simulink library "ddm"  (R2021b)
settings: Solver=VariableStepAuto  StartTime=0.0  StopTime=10.0  RelTol=1e-3
undefined symbols (not defined in the file or in its folder): ENUM_ADASACCSTA_ERROR, ENUM_ADASACCSTA_OFF, ENUM_ADASACCSTA_STANDBY, ENUM_ADASISASTA_OFF, ENUM_ALLOWMOV_ALLOWREADY, ENUM_APS, ENUM_BRKSTA_ERROR, ENUM_BRKSTA_OFF, ENUM_BRKSTA_ON, ENUM_CHGPREACTERRSTA_OBCPRE, ENUM_DCDCFAULTSTA_ANYFAULTLV1, ENUM_DCDCFAULTSTA_ANYFAULTLV2, ENUM_DRIVETRAIN_AWD, ENUM_DRIVETRAIN_FWD, ENUM_DRIVETRAIN_RWD, ENUM_DRSEATSTA_INVALID, ENUM_EDUDRTSTA_NORMAL, ENUM_EPBSTA_APPLIED, ENUM_EPBSTA_RELEASED, ENUM_HVBATTREADYPRE_READY, ENUM_MCUWARN_LV0, ENUM_MCUWARN_LV1, ENUM_MCUWARN_LV2, ENUM_MCUWARN_LV3, ENUM_MCUWARN_NOERROR, ENUM_OBCFAULTSTA_ANYFAULT, ENUM_PAS_R2F2, ENUM_PDFAULT_BATTPDFAIL, ENUM_PDFAULT_DCDCDISABLE, ENUM_PDFAULT_MCUDISABLE, ENUM_PDFAULT_MCUDISCHRG, ENUM_POWERSTA_OFF, ENUM_POWERSTA_ON, ENUM_POWERSTA_READY, ENUM_POWERSTA_STANDBY, ENUM_PRESSINDI_LOW, ENUM_PUFAULT_BATTUPFAIL, ENUM_PUFAULT_DCDCENABLEFAIL, ENUM_PUFAULT_PRECHRGCHKFAIL, ENUM_PUFAULT_SAFETYCHKFAIL, ENUM_PUSTATE_COMPLETED, ENUM_PWRSTASW_OFF, ENUM_PWRSTASW_OFFA, ENUM_PWRSTASW_OFFCHVCHRG, ENUM_PWRSTASW_OFFCLVCHRG, ENUM_PWRSTASW_ON, ENUM_PWRSTASW_ONHVCHRG, ENUM_PWRSTASW_READY, ENUM_PWRSTASW_STANDBY, ENUM_RANGESTA_12IN, ENUM_RANGESTA_12OUT, ENUM_SHIFTCOMMAND_D, ENUM_SHIFTCOMMAND_N, ENUM_SHIFTCOMMAND_P, ENUM_SHIFTCOMMAND_R, ENUM_ZONEMALFUNLV_1ST, ENUM_ZONEMALFUNLV_2ND, ENUM_ZONEMALFUNLV_3RD, ENUM_ZONEMALFUNLV_4TH, ENUM_ZONESPDCTRLMODE_ACC ... (+832)
libraries: hcu_lib x738, $bdroot x26, simulink x7
(part 19 of 25)

== system ddm/DDM/DDM/PMM/power up and power down/HVB ready for precharge fail ==
  note: Fail Safe Operation After Failure Decision
  note: Diagnostics and Fault Handling
  note: Release Condition After Failure Decision
  note: Fail Safe Operation During Failure Detection
  note: Test Pass Criteria
  note: Test Detection Criteria
  note: Release Condition During Failure Detection
  task_time_s : Inport
  VPMM_PowerSta_enum : Inport  Port=2
  VPMM_PwrStaSW_enum : Inport  Port=3
  VINP_HVBattReady4Pre_enum : Inport  Port=4
  VPMM_PowerUpFault_enum : Inport  Port=5
  DTC_clear_request : Inport  Port=6
  VPMM_PowerUpState_enum : Inport  Port=7
  Constant : Constant  Value=ENUM_PUFAULT_PRECHRGCHKFAIL
  Constant1 : Constant  Value=ENUM_PUSTATE_COMPLETED
  Constant10 : Constant  Value=KDDM_HVB4PreDTC_cnt
  Constant11 : Constant  Value=KDDM_HVB4PrePassSW_flg
  Constant15 : Constant  Value=KDDM_HVB4PreCFSSW_flg
  Constant16 : Constant  Value=TRUE
  Constant19 : Constant  Value=ENUM_POWERSTA_OFF
  Constant{2,21,25,27} (4 alike) : Constant  Value=FALSE
  Constant20 : Constant  Value=KDDM_HVB4PreDFSSW_flg
  Constant23 : Constant  Value=TRUE
  Constant24 : Constant  Value=TRUE
  Constant26 : Constant  Value=ENUM_PWRSTASW_OFF
  Constant3 : Constant  Value=ENUM_HVBATTREADYPRE_READY
  Constant38 : Constant  Commented=on  Value=KDDM_HVB4PreDetTO_s
  Constant40 : Constant  Commented=on  Value=KDDM_HVB4PreDTC_cnt
  Constant43 : Constant  Value=KDDM_HVB4PrePassTO_s
  Constant44 : Constant  Value=KDDM_HVB4PreDetSW_flg
  Constant8 : Constant  Value=KDDM_HVB4PrePassTO_s
  DTC_Couter : hcu_lib/Basic_Blocks/DTC_Couter
  DTC_Info : hcu_lib/Basic_Blocks/DTC_Info
  Data Type Conversion1 : DataTypeConversion  OutDataTypeStr=uint8
  Equal : RelationalOperator  Operator=~=  OutDataTypeStr=boolean  RndMeth=Simplest
  Equal1 : RelationalOperator  Operator===  OutDataTypeStr=boolean  RndMeth=Simplest
  Equal24 : RelationalOperator  Operator=~=  OutDataTypeStr=boolean  RndMeth=Simplest
  Equal4 : RelationalOperator  OutDataTypeStr=boolean  RndMeth=Simplest
  Equal5 : RelationalOperator  Operator===  OutDataTypeStr=boolean  RndMeth=Simplest
  Equal8 : RelationalOperator  Operator===  OutDataTypeStr=boolean  RndMeth=Simplest
  From48 : From  Commented=on  GotoTag=task_time_s
  Goto24 : Goto  Commented=on  GotoTag=VDDM_EDriveSysErrVCUErr_flg
  Logical Operator{4,12,15,18..19} (5 alike) : Logic  AllPortsSameDT=off  OutDataTypeStr=boolean
  Logical Operator3 : Logic  Operator=OR  AllPortsSameDT=off  OutDataTypeStr=boolean
  Logical Operator6 : Logic  Operator=NOT  AllPortsSameDT=off  OutDataTypeStr=boolean
  Logical Operator8 : Logic  Operator=OR  AllPortsSameDT=off  OutDataTypeStr=boolean
  Relay : Relay  OnSwitchValue=ONE_INT  OffSwitchValue=ZERO_INT
  SR_Latch1 : Subsystem  mask(SR_Latch){}
      mask help: SR latch function.
  SR_Latch3 : hcu_lib/Basic_Blocks/SR_Latch
  SR_Latch4 : hcu_lib/Basic_Blocks/SR_Latch
  Switch{,2,4..5} (4 alike) : Switch  Criteria=u2 ~= 0
  Test Detection Criteria : hcu_lib/Basic_Blocks/Test Detection Criteria  Commented=on
  Timer1 : hcu_lib/Basic_Blocks/Timer
  VDDM_HVB4PreDTC_raw32 : Outport
  wires:
  VPMM_PowerSta_enum/1 -> [VPMM_PowerSta_enum]
  VPMM_PwrStaSW_enum/1 -> [VPMM_PwrStaSW_enum]
  task_time_s/1 -> [task_time_s]
  Constant3/1 -> Equal24/2
  VINP_HVBattReady4Pre_enum/1 -> Equal24/1
  Logical Operator15/1 -> DTC_Couter/2
  Data Type Conversion1/1 -> [VDDM_HVB4PreDTC_cnt]  "VDDM_HVB4PreDTC_cnt"
  Constant11/1 -> Logical Operator15/2
  Constant40/1 -> Test Detection Criteria/3
  Constant43/1 -> Timer1/4
  Switch5/1 -> [VDDM_HVB4PreDet_flg]  "VDDM_HVB4PreDet_flg"
  Logical Operator3/1 -> Logical Operator15/1
  [VDDM_HVB4PreDTC_cnt] -> Relay/1
  [DTC_clear_request] -> Logical Operator8/2
  Constant23/1 -> Switch2/3
  Constant8/1 -> Equal4/2
  SR_Latch4/1 -> Logical Operator18/1
  Constant25/1 -> Switch4/3
  [VDDM_HVB4PreDet_flg] -> Logical Operator19/1
  Constant20/1 -> Logical Operator12/1
  Constant21/1 -> Switch/3
  Equal4/1 -> SR_Latch1/1(set)
  Switch4/1 -> [VDDM_HVB4PreCFSRls_flg]
  Constant26/1 -> Equal/2
  Logical Operator8/1 -> Switch4/2
  Constant16/1 -> Switch/1
  [VPMM_PowerSta_enum] -> Equal5/1
  Switch/1 -> Goto24/1
  SR_Latch3/1 -> Logical Operator12/2
  [VDDM_HVB4PreCFSRls_flg] -> Logical Operator3/2
  Logical Operator18/1 -> [VDDM_HVB4PreCFS_flg]
  DTC_Couter/2 -> Data Type Conversion1/1
  [VDDM_HVB4PrePass_flg] -> Logical Operator3/1
  Switch2/1 -> SR_Latch1/2(reset), Timer1/2, Logical Operator6/1
  Constant15/1 -> Logical Operator18/2
  Equal/1 -> Switch5/2
  Relay/1 -> SR_Latch3/1
  From48/1 -> Test Detection Criteria/2
  Logical Operator19/1 -> DTC_Couter/1
  [VDDM_HVB4PreCFS_flg] -> Switch/2
  [VPMM_PwrStaSW_enum] -> Equal/1
  Constant24/1 -> Switch4/1
  DTC_Couter/1 -> SR_Latch4/1
  SR_Latch1/1(latched) -> [VDDM_HVB4PrePass_flg]
  Logical Operator12/1 -> [VDDM_HVB4PreDFS_flg]
  Logical Operator6/1 -> Timer1/1
  Constant19/1 -> Equal5/2
  Constant27/1 -> Switch5/3
  Constant44/1 -> Logical Operator19/2
  Timer1/1 -> Equal4/1
  Equal5/1 -> Logical Operator8/1
  [VDDM_HVB4PreCFSRls_flg] -> SR_Latch4/2
  Constant10/1 -> DTC_Couter/3
  [VDDM_HVB4PreChk_flg] -> Switch5/1
  Constant1/1 -> Equal1/2
  Constant2/1 -> Switch2/1
  [VPMM_PowerUpState_enum] -> Equal1/1
  DTC_clear_request/1 -> [DTC_clear_request]
  Constant/1 -> Equal8/2
  VPMM_PowerUpFault_enum/1 -> Equal8/1
  Equal24/1 -> Logical Operator4/1
  Equal8/1 -> Logical Operator4/2
  Logical Operator4/1 -> [VDDM_HVB4PreChk_flg]
  [task_time_s] -> Timer1/3
  Equal1/1 -> Switch2/2
  DTC_Info/1 -> VDDM_HVB4PreDTC_raw32/1  "VDDM_HVB4PreDTC_raw32"
  [VDDM_HVB4PreCFS_flg] -> DTC_Info/3
  [VDDM_HVB4PreCFS_flg] -> SR_Latch3/2
  [VDDM_HVB4PrePass_flg] -> DTC_Info/2
  [VDDM_HVB4PreDet_flg] -> DTC_Info/1
  Constant38/1 -> Test Detection Criteria/4
  [DTC_clear_request] -> DTC_Info/4
  VPMM_PowerUpState_enum/1 -> [VPMM_PowerUpState_enum]

== system ddm/DDM/DDM/PMM/power up and power down/High level system safety check fail ==
  note: Fail Safe Operation After Failure Decision
  note: Fail Safe Operation During Failure Detection
  note: Diagnostics and Fault Handling
  note: Release Condition During Failure Detection
  note: Test Pass Criteria
  note: Test Detection Criteria
  note: Release Condition After Failure Decision
  task_time_s : Inport
  VPMM_PowerSta_enum : Inport  Port=2
  VPMM_PwrStaSW_enum : Inport  Port=3
  VPMM_SafetyChkHLv_flg : Inport  Port=4
  VPMM_PowerUpFault_enum : Inport  Port=5
  DTC_clear_request : Inport  Port=6
  VPMM_PowerUpState_enum : Inport  Port=7
  Constant : Constant  Value=ENUM_PUFAULT_SAFETYCHKFAIL
  Constant1 : Constant  Value=ENUM_PUSTATE_COMPLETED
  Constant10 : Constant  Value=KDDM_HiLvSaChkDTC_cnt
  Constant11 : Constant  Value=KDDM_HiLvSaChkPassSW_flg
  Constant15 : Constant  Value=KDDM_HiLvSaChkCFSSW_flg
  Constant16 : Constant  Value=TRUE
  Constant19 : Constant  Value=ENUM_POWERSTA_OFF
  Constant{2,21,25,27} (4 alike) : Constant  Value=FALSE
  Constant20 : Constant  Value=KDDM_HiLvSaChkDFSSW_flg
  Constant23 : Constant  Value=TRUE
  Constant24 : Constant  Value=TRUE
  Constant26 : Constant  Value=ENUM_PWRSTASW_OFF
  Constant38 : Constant  Commented=on  Value=KDDM_HiLvSaChkDetTO_s
  Constant40 : Constant  Commented=on  Value=KDDM_HiLvSaChkDTC_cnt
  Constant43 : Constant  Value=KDDM_HiLvSaChkPassTO_s
  Constant44 : Constant  Value=KDDM_HiLvSaChkDetSW_flg
  Constant8 : Constant  Value=KDDM_HiLvSaChkPassTO_s
  DTC_Couter : hcu_lib/Basic_Blocks/DTC_Couter
  DTC_Info : hcu_lib/Basic_Blocks/DTC_Info
  Data Type Conversion1 : DataTypeConversion  OutDataTypeStr=uint8
  Equal : RelationalOperator  Operator=~=  OutDataTypeStr=boolean  RndMeth=Simplest
  Equal1 : RelationalOperator  Operator===  OutDataTypeStr=boolean  RndMeth=Simplest
  Equal2 : RelationalOperator  Operator===  OutDataTypeStr=boolean  RndMeth=Simplest
  Equal5 : RelationalOperator  OutDataTypeStr=boolean  RndMeth=Simplest
  Equal6 : RelationalOperator  Operator===  OutDataTypeStr=boolean  RndMeth=Simplest
  From48 : From  Commented=on  GotoTag=task_time_s
  Goto24 : Goto  Commented=on  GotoTag=VDDM_EDriveSysErrVCUErr_flg
  Logical Operator{5,12,15,18..19} (5 alike) : Logic  AllPortsSameDT=off  OutDataTypeStr=boolean
  Logical Operator3 : Logic  Operator=OR  AllPortsSameDT=off  OutDataTypeStr=boolean
  Logical Operator4 : Logic  Operator=NOT  AllPortsSameDT=off  OutDataTypeStr=boolean
  Logical Operator6 : Logic  Operator=NOT  AllPortsSameDT=off  OutDataTypeStr=boolean
  Logical Operator8 : Logic  Operator=OR  AllPortsSameDT=off  OutDataTypeStr=boolean
  Relay : Relay  OnSwitchValue=ONE_INT  OffSwitchValue=ZERO_INT
  SR_Latch1 : Subsystem  mask(SR_Latch){}
      mask help: SR latch function.
  SR_Latch3 : hcu_lib/Basic_Blocks/SR_Latch
  SR_Latch4 : hcu_lib/Basic_Blocks/SR_Latch
  Switch{,2,4..5} (4 alike) : Switch  Criteria=u2 ~= 0
  Test Detection Criteria : hcu_lib/Basic_Blocks/Test Detection Criteria  Commented=on
  Timer1 : hcu_lib/Basic_Blocks/Timer
  VDDM_HiLvSaChkDTC_raw32 : Outport
  wires:
  Logical Operator5/1 -> [VDDM_HiLvSaChkChk_flg]
  VPMM_PowerUpFault_enum/1 -> Equal1/1
  VPMM_SafetyChkHLv_flg/1 -> Logical Operator4/1
  Logical Operator4/1 -> Logical Operator5/1
  Equal1/1 -> Logical Operator5/2
  Constant/1 -> Equal1/2
  DTC_clear_request/1 -> [DTC_clear_request]
  [VDDM_HiLvSaChkCFSRls_flg] -> SR_Latch4/2
  Switch2/1 -> Logical Operator6/1, Timer1/2, SR_Latch1/2(reset)
  Timer1/1 -> Equal5/1
  [VDDM_HiLvSaChkChk_flg] -> Switch5/1
  Constant19/1 -> Equal6/2
  Constant44/1 -> Logical Operator19/2
  DTC_Couter/2 -> Data Type Conversion1/1
  Constant43/1 -> Timer1/4
  Constant27/1 -> Switch5/3
  Equal6/1 -> Logical Operator8/1
  SR_Latch1/1(latched) -> [VDDM_HiLvSaChkPass_flg]
  Logical Operator6/1 -> Timer1/1
  Logical Operator8/1 -> Switch4/2
  Equal/1 -> Switch5/2
  Equal2/1 -> Switch2/2
  [VDDM_HiLvSaChkDTC_cnt] -> Relay/1
  Constant11/1 -> Logical Operator15/2
  [DTC_clear_request] -> Logical Operator8/2
  [VDDM_HiLvSaChkCFS_flg] -> Switch/2
  Relay/1 -> SR_Latch3/1
  [VPMM_PwrStaSW_enum] -> Equal/1
  Constant25/1 -> Switch4/3
  Constant40/1 -> Test Detection Criteria/3
  Constant10/1 -> DTC_Couter/3
  Logical Operator15/1 -> DTC_Couter/2
  SR_Latch4/1 -> Logical Operator18/1
  Constant24/1 -> Switch4/1
  Logical Operator3/1 -> Logical Operator15/1
  [VDDM_HiLvSaChkDet_flg] -> Logical Operator19/1
  Switch5/1 -> [VDDM_HiLvSaChkDet_flg]  "VDDM_HiLvSaChkDet_flg"
  Switch/1 -> Goto24/1
  From48/1 -> Test Detection Criteria/2
  SR_Latch3/1 -> Logical Operator12/2
  Constant26/1 -> Equal/2
  Constant16/1 -> Switch/1
  Constant23/1 -> Switch2/3
  [VDDM_HiLvSaChkPass_flg] -> Logical Operator3/1
  [VPMM_PowerSta_enum] -> Equal6/1
  Logical Operator19/1 -> DTC_Couter/1
  [VDDM_HiLvSaChkCFSRls_flg] -> Logical Operator3/2
  DTC_Couter/1 -> SR_Latch4/1
  [task_time_s] -> Timer1/3
  Constant15/1 -> Logical Operator18/2
  Logical Operator12/1 -> [VDDM_HiLvSaChkDFS_flg]
  Constant20/1 -> Logical Operator12/1
  Constant8/1 -> Equal5/2
  Data Type Conversion1/1 -> [VDDM_HiLvSaChkDTC_cnt]  "VDDM_HiLvSaChkDTC_cnt"
  Switch4/1 -> [VDDM_HiLvSaChkCFSRls_flg]
  Equal5/1 -> SR_Latch1/1(set)
  Constant21/1 -> Switch/3
  Logical Operator18/1 -> [VDDM_HiLvSaChkCFS_flg]
  VPMM_PowerSta_enum/1 -> [VPMM_PowerSta_enum]
  VPMM_PwrStaSW_enum/1 -> [VPMM_PwrStaSW_enum]
  task_time_s/1 -> [task_time_s]
  DTC_Info/1 -> VDDM_HiLvSaChkDTC_raw32/1  "VDDM_HiLvSaChkDTC_raw32"
  [VDDM_HiLvSaChkPass_flg] -> DTC_Info/2
  [VDDM_HiLvSaChkCFS_flg] -> DTC_Info/3
  [VDDM_HiLvSaChkCFS_flg] -> SR_Latch3/2
  [VDDM_HiLvSaChkDet_flg] -> DTC_Info/1
  Constant38/1 -> Test Detection Criteria/4
  [DTC_clear_request] -> DTC_Info/4
  VPMM_PowerUpState_enum/1 -> [VPMM_PowerUpState_enum]
  Constant2/1 -> Switch2/1
  Constant1/1 -> Equal2/2
  [VPMM_PowerUpState_enum] -> Equal2/1

== system ddm/DDM/DDM/PMM/power up and power down/MCU active discharge fail ==
  note: Release Condition During Failure Detection
  note: Fail Safe Operation After Failure Decision
  note: Fail Safe Operation During Failure Detection
  note: Test Detection Criteria
  note: Diagnostics and Fault Handling
  note: Test Pass Criteria
  note: Release Condition After Failure Decision
  task_time_s : Inport
  VPMM_PowerSta_enum : Inport  Port=2
  VPMM_PwrStaSW_enum : Inport  Port=3
  VPMM_PowerDownFault_enum : Inport  Port=4
  DTC_clear_request : Inport  Port=5
  Constant : Constant  Value=ENUM_PDFAULT_MCUDISCHRG
  Constant1 : Constant  Value=ENUM_PWRSTASW_OFF
  Constant10 : Constant  Value=KDDM_MCUActDTC_cnt
  Constant11 : Constant  Value=KDDM_MCUActPassSW_flg
  Constant15 : Constant  Value=KDDM_MCUActCFSSW_flg
  Constant16 : Constant  Value=TRUE
  Constant17 : Constant  Value=KDDM_MCUActPassTO_s
  Constant19 : Constant  Value=ENUM_POWERSTA_OFF
  Constant20 : Constant  Value=KDDM_MCUActDFSSW_flg
  Constant21 : Constant  Value=FALSE
  Constant22 : Constant  Value=ENUM_PWRSTASW_OFF
  Constant23 : Constant  Value=TRUE
  Constant24 : Constant  Value=TRUE
  Constant25 : Constant  Value=FALSE
  Constant27 : Constant  Value=FALSE
  Constant38 : Constant  Commented=on  Value=KDDM_MCUActDetTO_s
  Constant40 : Constant  Commented=on  Value=KDDM_MCUActDTC_cnt
  Constant43 : Constant  Value=KDDM_MCUActPassTO_s
  Constant44 : Constant  Value=KDDM_MCUActDetSW_flg
  DTC_Couter : hcu_lib/Basic_Blocks/DTC_Couter
  DTC_Info : hcu_lib/Basic_Blocks/DTC_Info
  Data Type Conversion1 : DataTypeConversion  OutDataTypeStr=uint8
  Equal1 : RelationalOperator  Operator===  OutDataTypeStr=boolean  RndMeth=Simplest
  Equal2 : RelationalOperator  Operator=~=  OutDataTypeStr=boolean  RndMeth=Simplest
  Equal4 : RelationalOperator  Operator=~=  OutDataTypeStr=boolean  RndMeth=Simplest
  Equal6 : RelationalOperator  OutDataTypeStr=boolean  RndMeth=Simplest
  Equal7 : RelationalOperator  Operator===  OutDataTypeStr=boolean  RndMeth=Simplest
  From48 : From  Commented=on  GotoTag=task_time_s
  Logical Operator{12,15,18..19} (4 alike) : Logic  AllPortsSameDT=off  OutDataTypeStr=boolean
  Logical Operator3 : Logic  Operator=OR  AllPortsSameDT=off  OutDataTypeStr=boolean
  Logical Operator6 : Logic  Operator=NOT  AllPortsSameDT=off  OutDataTypeStr=boolean
  Logical Operator8 : Logic  Operator=OR  AllPortsSameDT=off  OutDataTypeStr=boolean
  Relay : Relay  OnSwitchValue=ONE_INT  OffSwitchValue=ZERO_INT
  SR_Latch1 : Subsystem  mask(SR_Latch){}
      mask help: SR latch function.
  SR_Latch3 : hcu_lib/Basic_Blocks/SR_Latch
  SR_Latch4 : hcu_lib/Basic_Blocks/SR_Latch
  Switch{,1,4..5} (4 alike) : Switch  Criteria=u2 ~= 0
  Test Detection Criteria : hcu_lib/Basic_Blocks/Test Detection Criteria  Commented=on
  Timer1 : hcu_lib/Basic_Blocks/Timer
  VDDM_MCUActDTC_raw32 : Outport
  VDDM_MCUActDisFail_flg : Outport  Port=2
  wires:
  VPMM_PowerSta_enum/1 -> [VPMM_PowerSta_enum]
  VPMM_PwrStaSW_enum/1 -> [VPMM_PwrStaSW_enum]
  task_time_s/1 -> [task_time_s]
  DTC_Couter/1 -> SR_Latch4/1
  Constant27/1 -> Switch5/3
  Constant23/1 -> Switch1/3
  SR_Latch4/1 -> Logical Operator18/1
  Constant11/1 -> Logical Operator15/2
  [VPMM_PowerSta_enum] -> Equal7/1
  Logical Operator15/1 -> DTC_Couter/2
  Constant20/1 -> Logical Operator12/1
  Equal2/1 -> Switch1/2
  [VDDM_MCUActDTC_cnt] -> Relay/1
  SR_Latch1/1(latched) -> [VDDM_MCUActPass_flg]
  Equal4/1 -> Switch5/2
  [VPMM_PwrStaSW_enum] -> Equal2/1
  Logical Operator12/1 -> [VDDM_MCUActDFS_flg]
  Constant1/1 -> Equal2/2
  Switch5/1 -> [VDDM_MCUActDet_flg]  "VDDM_MCUActDet_flg"
  Constant15/1 -> Logical Operator18/2
  [DTC_clear_request] -> Logical Operator8/2
  Constant40/1 -> Test Detection Criteria/3
  Switch4/1 -> [VDDM_MCUActCFSRls_flg]
  From48/1 -> Test Detection Criteria/2
  [VDDM_MCUActCFSRls_flg] -> Logical Operator3/2
  DTC_Couter/2 -> Data Type Conversion1/1
  SR_Latch3/1 -> Logical Operator12/2
  Constant17/1 -> Equal6/2
  Data Type Conversion1/1 -> [VDDM_MCUActDTC_cnt]  "VDDM_MCUActDTC_cnt"
  Logical Operator6/1 -> Timer1/1
  Switch/1 -> [VDDM_MCUActDisFail_flg]  "VDDM_MCUActDisFail_flg"
  Constant24/1 -> Switch4/1
  Constant16/1 -> Switch/1
  Timer1/1 -> Equal6/1
  Logical Operator18/1 -> [VDDM_MCUActCFS_flg]
  Switch1/1 -> Logical Operator6/1, SR_Latch1/2(reset), Timer1/2
  Constant10/1 -> DTC_Couter/3
  Logical Operator19/1 -> DTC_Couter/1
  Equal6/1 -> SR_Latch1/1(set)
  Constant44/1 -> Logical Operator19/2
  Constant43/1 -> Timer1/4
  Relay/1 -> SR_Latch3/1
  Logical Operator8/1 -> Switch4/2
  Constant22/1 -> Equal4/2
  Constant25/1 -> Switch4/3
  Equal7/1 -> Logical Operator8/1
  [VDDM_MCUActChk_flg] -> Switch1/1
  [VDDM_MCUActCFSRls_flg] -> SR_Latch4/2
  [VDDM_MCUActCFS_flg] -> Switch/2
  [task_time_s] -> Timer1/3
  Constant21/1 -> Switch/3
  [VPMM_PwrStaSW_enum] -> Equal4/1
  Logical Operator3/1 -> Logical Operator15/1
  [VDDM_MCUActPass_flg] -> Logical Operator3/1
  [VDDM_MCUActDet_flg] -> Logical Operator19/1
  Constant19/1 -> Equal7/2
  [VDDM_MCUActChk_flg] -> Switch5/1
  DTC_clear_request/1 -> [DTC_clear_request]
  Constant/1 -> Equal1/2
  VPMM_PowerDownFault_enum/1 -> Equal1/1
  Equal1/1 -> [VDDM_MCUActChk_flg]
  [VDDM_MCUActDisFail_flg] -> VDDM_MCUActDisFail_flg/1
  DTC_Info/1 -> VDDM_MCUActDTC_raw32/1  "VDDM_MCUActDTC_raw32"
  [VDDM_MCUActPass_flg] -> DTC_Info/2
  [VDDM_MCUActCFS_flg] -> DTC_Info/3
  [VDDM_MCUActCFS_flg] -> SR_Latch3/2
  [VDDM_MCUActDet_flg] -> DTC_Info/1
  Constant38/1 -> Test Detection Criteria/4
  [DTC_clear_request] -> DTC_Info/4

== system ddm/DDM/DDM/PMM/power up and power down/MCU disable fail ==
  note: Test Pass Criteria
  note: Release Condition After Failure Decision
  note: Test Detection Criteria
  note: Fail Safe Operation During Failure Detection
  note: Diagnostics and Fault Handling
  note: Release Condition During Failure Detection
  note: Fail Safe Operation After Failure Decision
  task_time_s : Inport
  VPMM_PowerSta_enum : Inport  Port=2
  VPMM_PwrStaSW_enum : Inport  Port=3
  VPMM_PowerDownFault_enum : Inport  Port=4
  DTC_clear_request : Inport  Port=5
  Constant : Constant  Value=ENUM_PDFAULT_MCUDISABLE
  Constant10 : Constant  Value=KDDM_MCUDisDTC_cnt
  Constant11 : Constant  Value=KDDM_MCUDisPassSW_flg
  Constant15 : Constant  Value=KDDM_MCUDisCFSSW_flg
  Constant16 : Constant  Value=TRUE
  Constant17 : Constant  Value=KDDM_MCUDisPassTO_s
  Constant19 : Constant  Value=ENUM_POWERSTA_OFF
  Constant2 : Constant  Value=ENUM_PWRSTASW_OFF
  Constant20 : Constant  Value=KDDM_MCUDisDFSSW_flg
  Constant21 : Constant  Value=FALSE
  Constant22 : Constant  Value=ENUM_PWRSTASW_OFF
  Constant23 : Constant  Value=TRUE
  Constant24 : Constant  Value=TRUE
  Constant25 : Constant  Value=FALSE
  Constant27 : Constant  Value=FALSE
  Constant38 : Constant  Commented=on  Value=KDDM_MCUDisDetTO_s
  Constant40 : Constant  Commented=on  Value=KDDM_MCUDisDTC_cnt
  Constant43 : Constant  Value=KDDM_MCUDisPassTO_s
  Constant44 : Constant  Value=KDDM_MCUDisDetSW_flg
  DTC_Couter : hcu_lib/Basic_Blocks/DTC_Couter
  DTC_Info : hcu_lib/Basic_Blocks/DTC_Info
  Data Type Conversion1 : DataTypeConversion  OutDataTypeStr=uint8
  Equal1 : RelationalOperator  Operator===  OutDataTypeStr=boolean  RndMeth=Simplest
  Equal2 : RelationalOperator  Operator=~=  OutDataTypeStr=boolean  RndMeth=Simplest
  Equal4 : RelationalOperator  Operator=~=  OutDataTypeStr=boolean  RndMeth=Simplest
  Equal6 : RelationalOperator  OutDataTypeStr=boolean  RndMeth=Simplest
  Equal7 : RelationalOperator  Operator===  OutDataTypeStr=boolean  RndMeth=Simplest
  From48 : From  Commented=on  GotoTag=task_time_s
  Goto24 : Goto  Commented=on  GotoTag=VDDM_EDriveSysErrVCUErr_flg
  Logical Operator{12,15,18..19} (4 alike) : Logic  AllPortsSameDT=off  OutDataTypeStr=boolean
  Logical Operator3 : Logic  Operator=OR  AllPortsSameDT=off  OutDataTypeStr=boolean
  Logical Operator6 : Logic  Operator=NOT  AllPortsSameDT=off  OutDataTypeStr=boolean
  Logical Operator8 : Logic  Operator=OR  AllPortsSameDT=off  OutDataTypeStr=boolean
  Relay : Relay  OnSwitchValue=ONE_INT  OffSwitchValue=ZERO_INT
  SR_Latch1 : Subsystem  mask(SR_Latch){}
      mask help: SR latch function.
  SR_Latch3 : hcu_lib/Basic_Blocks/SR_Latch
  SR_Latch4 : hcu_lib/Basic_Blocks/SR_Latch
  Switch{,1,4..5} (4 alike) : Switch  Criteria=u2 ~= 0
  Test Detection Criteria : hcu_lib/Basic_Blocks/Test Detection Criteria  Commented=on
  Timer1 : hcu_lib/Basic_Blocks/Timer
  VDDM_MCUDisDTC_raw32 : Outport
  wires:
  task_time_s/1 -> [task_time_s]
  VPMM_PwrStaSW_enum/1 -> [VPMM_PwrStaSW_enum]
  VPMM_PowerSta_enum/1 -> [VPMM_PowerSta_enum]
  Constant23/1 -> Switch1/3
  [VDDM_MCUDisChk_flg] -> Switch1/1
  Equal2/1 -> Switch1/2
  Equal4/1 -> Switch5/2
  Switch1/1 -> Logical Operator6/1, SR_Latch1/2(reset), Timer1/2
  DTC_Couter/2 -> Data Type Conversion1/1
  SR_Latch4/1 -> Logical Operator18/1
  [VPMM_PowerSta_enum] -> Equal7/1
  [VPMM_PwrStaSW_enum] -> Equal4/1
  Constant17/1 -> Equal6/2
  Logical Operator15/1 -> DTC_Couter/2
  Constant11/1 -> Logical Operator15/2
  [VDDM_MCUDisPass_flg] -> Logical Operator3/1
  Constant43/1 -> Timer1/4
  Logical Operator19/1 -> DTC_Couter/1
  DTC_Couter/1 -> SR_Latch4/1
  [VDDM_MCUDisCFSRls_flg] -> SR_Latch4/2
  Constant27/1 -> Switch5/3
  Constant25/1 -> Switch4/3
  Constant16/1 -> Switch/1
  [VDDM_MCUDisChk_flg] -> Switch5/1
  [VDDM_MCUDisCFS_flg] -> Switch/2
  Switch4/1 -> [VDDM_MCUDisCFSRls_flg]
  Constant19/1 -> Equal7/2
  Data Type Conversion1/1 -> [VDDM_MCUDisDTC_cnt]  "VDDM_MCUDisDTC_cnt"
  Logical Operator3/1 -> Logical Operator15/1
  [VDDM_MCUDisDet_flg] -> Logical Operator19/1
  Equal6/1 -> SR_Latch1/1(set)
  Constant21/1 -> Switch/3
  Constant15/1 -> Logical Operator18/2
  Logical Operator18/1 -> [VDDM_MCUDisCFS_flg]
  Switch/1 -> Goto24/1
  Logical Operator12/1 -> [VDDM_MCUDisDFS_flg]
  SR_Latch3/1 -> Logical Operator12/2
  From48/1 -> Test Detection Criteria/2
  Equal7/1 -> Logical Operator8/1
  Constant44/1 -> Logical Operator19/2
  [VDDM_MCUDisCFSRls_flg] -> Logical Operator3/2
  Logical Operator8/1 -> Switch4/2
  Constant24/1 -> Switch4/1
  Switch5/1 -> [VDDM_MCUDisDet_flg]  "VDDM_MCUDisDet_flg"
  Logical Operator6/1 -> Timer1/1
  SR_Latch1/1(latched) -> [VDDM_MCUDisPass_flg]
  [VDDM_MCUDisDTC_cnt] -> Relay/1
  Relay/1 -> SR_Latch3/1
  Constant20/1 -> Logical Operator12/1
  Constant22/1 -> Equal4/2
  [DTC_clear_request] -> Logical Operator8/2
  Constant40/1 -> Test Detection Criteria/3
  [task_time_s] -> Timer1/3
  Timer1/1 -> Equal6/1
  Constant10/1 -> DTC_Couter/3
  Constant/1 -> Equal1/2
  VPMM_PowerDownFault_enum/1 -> Equal1/1
  DTC_clear_request/1 -> [DTC_clear_request]
  [VPMM_PwrStaSW_enum] -> Equal2/1
  Constant2/1 -> Equal2/2
  Equal1/1 -> [VDDM_MCUDisChk_flg]
  DTC_Info/1 -> VDDM_MCUDisDTC_raw32/1  "VDDM_MCUDisDTC_raw32"
  [VDDM_MCUDisPass_flg] -> DTC_Info/2
  [VDDM_MCUDisCFS_flg] -> DTC_Info/3
  [VDDM_MCUDisCFS_flg] -> SR_Latch3/2
  [VDDM_MCUDisDet_flg] -> DTC_Info/1
  Constant38/1 -> Test Detection Criteria/4
  [DTC_clear_request] -> DTC_Info/4

== system ddm/DDM/DDM/PMM/power up and power down/MCU ready for precharge fail ==
  note: Test Pass Criteria
  note: Fail Safe Operation During Failure Detection
  note: Test Detection Criteria
  note: Release Condition During Failure Detection
  note: Release Condition After Failure Decision
  note: Fail Safe Operation After Failure Decision
  note: Diagnostics and Fault Handling
  task_time_s : Inport
  VPMM_PowerSta_enum : Inport  Port=2
  VPMM_PwrStaSW_enum : Inport  Port=3
  VPMM_MCUReady4Pre_flg : Inport  Port=4
  VPMM_PowerUpFault_enum : Inport  Port=5
  DTC_clear_request : Inport  Port=6
  VPMM_PowerUpState_enum : Inport  Port=7
  Constant : Constant  Value=ENUM_PUFAULT_PRECHRGCHKFAIL
  Constant1 : Constant  Value=ENUM_PUSTATE_COMPLETED
  Constant10 : Constant  Value=KDDM_MCU4PreDTC_cnt
  Constant11 : Constant  Value=KDDM_MCU4PrePassSW_flg
  Constant15 : Constant  Value=KDDM_MCU4PreCFSSW_flg
  Constant16 : Constant  Value=TRUE
  Constant19 : Constant  Value=ENUM_POWERSTA_OFF
  Constant{2,21,25,27} (4 alike) : Constant  Value=FALSE
  Constant20 : Constant  Value=KDDM_MCU4PreDFSSW_flg
  Constant23 : Constant  Value=TRUE
  Constant24 : Constant  Value=TRUE
  Constant26 : Constant  Value=ENUM_PWRSTASW_OFF
  Constant38 : Constant  Commented=on  Value=KDDM_MCU4PreDetTO_s
  Constant40 : Constant  Commented=on  Value=KDDM_MCU4PreDTC_cnt
  Constant43 : Constant  Value=KDDM_MCU4PrePassTO_s
  Constant44 : Constant  Value=KDDM_MCU4PreDetSW_flg
  Constant8 : Constant  Value=KDDM_MCU4PrePassTO_s
  DTC_Couter : hcu_lib/Basic_Blocks/DTC_Couter
  DTC_Info : hcu_lib/Basic_Blocks/DTC_Info
  Data Type Conversion1 : DataTypeConversion  OutDataTypeStr=uint8
  Equal : RelationalOperator  Operator=~=  OutDataTypeStr=boolean  RndMeth=Simplest
  Equal1 : RelationalOperator  Operator===  OutDataTypeStr=boolean  RndMeth=Simplest
  Equal2 : RelationalOperator  Operator===  OutDataTypeStr=boolean  RndMeth=Simplest
  Equal5 : RelationalOperator  OutDataTypeStr=boolean  RndMeth=Simplest
  Equal6 : RelationalOperator  Operator===  OutDataTypeStr=boolean  RndMeth=Simplest
  From48 : From  Commented=on  GotoTag=task_time_s
  Goto24 : Goto  Commented=on  GotoTag=VDDM_EDriveSysErrVCUErr_flg
  Logical Operator{4,12,15,18..19} (5 alike) : Logic  AllPortsSameDT=off  OutDataTypeStr=boolean
  Logical Operator3 : Logic  Operator=OR  AllPortsSameDT=off  OutDataTypeStr=boolean
  Logical Operator5 : Logic  Operator=NOT  AllPortsSameDT=off  OutDataTypeStr=boolean
  Logical Operator6 : Logic  Operator=NOT  AllPortsSameDT=off  OutDataTypeStr=boolean
  Logical Operator8 : Logic  Operator=OR  AllPortsSameDT=off  OutDataTypeStr=boolean
  Relay : Relay  OnSwitchValue=ONE_INT  OffSwitchValue=ZERO_INT
  SR_Latch1 : Subsystem  mask(SR_Latch){}
      mask help: SR latch function.
  SR_Latch3 : hcu_lib/Basic_Blocks/SR_Latch
  SR_Latch4 : hcu_lib/Basic_Blocks/SR_Latch
  Switch{,2,4..5} (4 alike) : Switch  Criteria=u2 ~= 0
  Test Detection Criteria : hcu_lib/Basic_Blocks/Test Detection Criteria  Commented=on
  Timer1 : hcu_lib/Basic_Blocks/Timer
  VDDM_MCU4PreDTC_raw32 : Outport
  wires:
  task_time_s/1 -> [task_time_s]
  VPMM_PwrStaSW_enum/1 -> [VPMM_PwrStaSW_enum]
  VPMM_PowerSta_enum/1 -> [VPMM_PowerSta_enum]
  [task_time_s] -> Timer1/3
  Equal2/1 -> Switch2/2
  Logical Operator19/1 -> DTC_Couter/1
  From48/1 -> Test Detection Criteria/2
  [VDDM_MCU4PreCFSRls_flg] -> Logical Operator3/2
  [VDDM_MCU4PrePass_flg] -> Logical Operator3/1
  [VPMM_PowerSta_enum] -> Equal6/1
  Logical Operator18/1 -> [VDDM_MCU4PreCFS_flg]
  SR_Latch3/1 -> Logical Operator12/2
  Switch/1 -> Goto24/1
  Constant16/1 -> Switch/1
  Constant26/1 -> Equal/2
  Switch4/1 -> [VDDM_MCU4PreCFSRls_flg]
  Equal5/1 -> SR_Latch1/1(set)
  Constant20/1 -> Logical Operator12/1
  Constant15/1 -> Logical Operator18/2
  Constant21/1 -> Switch/3
  Constant25/1 -> Switch4/3
  SR_Latch4/1 -> Logical Operator18/1
  Constant8/1 -> Equal5/2
  Constant24/1 -> Switch4/1
  Constant40/1 -> Test Detection Criteria/3
  Constant43/1 -> Timer1/4
  [VPMM_PwrStaSW_enum] -> Equal/1
  Logical Operator3/1 -> Logical Operator15/1
  [VDDM_MCU4PreDet_flg] -> Logical Operator19/1
  Switch5/1 -> [VDDM_MCU4PreDet_flg]  "VDDM_MCU4PreDet_flg"
  [DTC_clear_request] -> Logical Operator8/2
  [VDDM_MCU4PreCFS_flg] -> Switch/2
  Equal/1 -> Switch5/2
  [VDDM_MCU4PreDTC_cnt] -> Relay/1
  Relay/1 -> SR_Latch3/1
  Constant11/1 -> Logical Operator15/2
  Data Type Conversion1/1 -> [VDDM_MCU4PreDTC_cnt]  "VDDM_MCU4PreDTC_cnt"
  Logical Operator8/1 -> Switch4/2
  Constant27/1 -> Switch5/3
  DTC_Couter/2 -> Data Type Conversion1/1
  Constant44/1 -> Logical Operator19/2
  DTC_Couter/1 -> SR_Latch4/1
  Logical Operator6/1 -> Timer1/1
  Constant19/1 -> Equal6/2
  Constant23/1 -> Switch2/3
  Logical Operator12/1 -> [VDDM_MCU4PreDFS_flg]
  Constant10/1 -> DTC_Couter/3
  Logical Operator15/1 -> DTC_Couter/2
  Equal6/1 -> Logical Operator8/1
  SR_Latch1/1(latched) -> [VDDM_MCU4PrePass_flg]
  [VDDM_MCU4PreChk_flg] -> Switch5/1
  Timer1/1 -> Equal5/1
  Switch2/1 -> SR_Latch1/2(reset), Timer1/2, Logical Operator6/1
  [VDDM_MCU4PreCFSRls_flg] -> SR_Latch4/2
  DTC_clear_request/1 -> [DTC_clear_request]
  Constant/1 -> Equal1/2
  VPMM_PowerUpFault_enum/1 -> Equal1/1
  Logical Operator5/1 -> Logical Operator4/1
  Equal1/1 -> Logical Operator4/2
  Logical Operator4/1 -> [VDDM_MCU4PreChk_flg]
  VPMM_MCUReady4Pre_flg/1 -> Logical Operator5/1
  [VDDM_MCU4PrePass_flg] -> DTC_Info/2
  DTC_Info/1 -> VDDM_MCU4PreDTC_raw32/1  "VDDM_MCU4PreDTC_raw32"
  [VDDM_MCU4PreCFS_flg] -> DTC_Info/3
  [VDDM_MCU4PreCFS_flg] -> SR_Latch3/2
  [VDDM_MCU4PreDet_flg] -> DTC_Info/1
  Constant38/1 -> Test Detection Criteria/4
  [DTC_clear_request] -> DTC_Info/4
  VPMM_PowerUpState_enum/1 -> [VPMM_PowerUpState_enum]
  Constant2/1 -> Switch2/1
  Constant1/1 -> Equal2/2
  [VPMM_PowerUpState_enum] -> Equal2/1

== system ddm/DDM/DDM/PMM/power up and power down/Mid level system safety check fail ==
  note: Diagnostics and Fault Handling
  note: Test Pass Criteria
  note: Release Condition During Failure Detection
  note: Fail Safe Operation During Failure Detection
  note: Fail Safe Operation After Failure Decision
  note: Release Condition After Failure Decision
  note: Test Detection Criteria
  task_time_s : Inport
  VPMM_PowerSta_enum : Inport  Port=2
  VPMM_PwrStaSW_enum : Inport  Port=3
  VDDM_MidLvSaChkChk_flg : Inport  Port=4
  VPMM_PowerUpFault_enum : Inport  Port=5
  DTC_clear_request : Inport  Port=6
  VPMM_PowerUpState_enum : Inport  Port=7
  Constant : Constant  Value=ENUM_PUFAULT_SAFETYCHKFAIL
  Constant1 : Constant  Value=ENUM_PUSTATE_COMPLETED
  Constant10 : Constant  Value=KDDM_MidLvSaChkDTC_cnt
  Constant11 : Constant  Value=KDDM_MidLvSaChkPassSW_flg
  Constant15 : Constant  Value=KDDM_MidLvSaChkCFSSW_flg
  Constant16 : Constant  Value=TRUE
  Constant19 : Constant  Value=ENUM_POWERSTA_OFF
  Constant{2,21,25,27} (4 alike) : Constant  Value=FALSE
  Constant20 : Constant  Value=KDDM_MidLvSaChkDFSSW_flg
  Constant23 : Constant  Value=TRUE
  Constant24 : Constant  Value=TRUE
  Constant26 : Constant  Value=ENUM_PWRSTASW_OFF
  Constant38 : Constant  Commented=on  Value=KDDM_MidLvSaChkDetTO_s
  Constant40 : Constant  Commented=on  Value=KDDM_MidLvSaChkDTC_cnt
  Constant43 : Constant  Value=KDDM_MidLvSaChkPassTO_s
  Constant44 : Constant  Value=KDDM_MidLvSaChkDetSW_flg
  Constant8 : Constant  Value=KDDM_MidLvSaChkPassTO_s
  DTC_Couter : hcu_lib/Basic_Blocks/DTC_Couter
  DTC_Info : hcu_lib/Basic_Blocks/DTC_Info
  Data Type Conversion1 : DataTypeConversion  OutDataTypeStr=uint8
  Equal : RelationalOperator  Operator=~=  OutDataTypeStr=boolean  RndMeth=Simplest
  Equal1 : RelationalOperator  Operator===  OutDataTypeStr=boolean  RndMeth=Simplest
  Equal2 : RelationalOperator  Operator===  OutDataTypeStr=boolean  RndMeth=Simplest
  Equal5 : RelationalOperator  OutDataTypeStr=boolean  RndMeth=Simplest
  Equal6 : RelationalOperator  Operator===  OutDataTypeStr=boolean  RndMeth=Simplest
  From48 : From  Commented=on  GotoTag=task_time_s
  Goto24 : Goto  Commented=on  GotoTag=VDDM_EDriveSysErrVCUErr_flg
  Logical Operator{5,12,15,18..19} (5 alike) : Logic  AllPortsSameDT=off  OutDataTypeStr=boolean
  Logical Operator3 : Logic  Operator=OR  AllPortsSameDT=off  OutDataTypeStr=boolean
  Logical Operator4 : Logic  Operator=NOT  AllPortsSameDT=off  OutDataTypeStr=boolean
  Logical Operator6 : Logic  Operator=NOT  AllPortsSameDT=off  OutDataTypeStr=boolean
  Logical Operator8 : Logic  Operator=OR  AllPortsSameDT=off  OutDataTypeStr=boolean
  Relay : Relay  OnSwitchValue=ONE_INT  OffSwitchValue=ZERO_INT
  SR_Latch1 : Subsystem  mask(SR_Latch){}
      mask help: SR latch function.
  SR_Latch3 : hcu_lib/Basic_Blocks/SR_Latch
  SR_Latch4 : hcu_lib/Basic_Blocks/SR_Latch
  Switch{,2,4..5} (4 alike) : Switch  Criteria=u2 ~= 0
  Test Detection Criteria : hcu_lib/Basic_Blocks/Test Detection Criteria  Commented=on
  Timer1 : hcu_lib/Basic_Blocks/Timer
  VDDM_MidLvSaChkDTC_raw32 : Outport
  wires:
  VPMM_PowerSta_enum/1 -> [VPMM_PowerSta_enum]
  VPMM_PwrStaSW_enum/1 -> [VPMM_PwrStaSW_enum]
  task_time_s/1 -> [task_time_s]
  Constant44/1 -> Logical Operator19/2
  Data Type Conversion1/1 -> [VDDM_MidLvSaChkDTC_cnt]  "VDDM_MidLvSaChkDTC_cnt"
  Constant16/1 -> Switch/1
  [VDDM_MidLvSaChkChk_flg] -> Switch5/1
  Constant8/1 -> Equal5/2
  Constant19/1 -> Equal6/2
  [VPMM_PwrStaSW_enum] -> Equal/1
  Logical Operator18/1 -> [VDDM_MidLvSaChkCFS_flg]
  Switch4/1 -> [VDDM_MidLvSaChkCFSRls_flg]
  Constant21/1 -> Switch/3
  [VDDM_MidLvSaChkCFS_flg] -> Switch/2
  Constant20/1 -> Logical Operator12/1
  Equal2/1 -> Switch2/2
  Logical Operator12/1 -> [VDDM_MidLvSaChkDFS_flg]
  Equal6/1 -> Logical Operator8/1
  Equal5/1 -> SR_Latch1/1(set)
  Constant15/1 -> Logical Operator18/2
  From48/1 -> Test Detection Criteria/2
  SR_Latch3/1 -> Logical Operator12/2
  Constant23/1 -> Switch2/3
  Switch/1 -> Goto24/1
  Switch5/1 -> [VDDM_MidLvSaChkDet_flg]  "VDDM_MidLvSaChkDet_flg"
  Constant25/1 -> Switch4/3
  Logical Operator6/1 -> Timer1/1
  SR_Latch1/1(latched) -> [VDDM_MidLvSaChkPass_flg]
  Constant26/1 -> Equal/2
  [VDDM_MidLvSaChkCFSRls_flg] -> Logical Operator3/2
  Constant43/1 -> Timer1/4
  Constant24/1 -> Switch4/1
  [VDDM_MidLvSaChkDTC_cnt] -> Relay/1
  Constant10/1 -> DTC_Couter/3
  Relay/1 -> SR_Latch3/1
  SR_Latch4/1 -> Logical Operator18/1
  Constant11/1 -> Logical Operator15/2
  [DTC_clear_request] -> Logical Operator8/2
  Logical Operator3/1 -> Logical Operator15/1
  [VDDM_MidLvSaChkDet_flg] -> Logical Operator19/1
  [VPMM_PowerSta_enum] -> Equal6/1
  Logical Operator19/1 -> DTC_Couter/1
  Logical Operator15/1 -> DTC_Couter/2
  Equal/1 -> Switch5/2
  Constant27/1 -> Switch5/3
  [VDDM_MidLvSaChkPass_flg] -> Logical Operator3/1
  [VDDM_MidLvSaChkCFSRls_flg] -> SR_Latch4/2
  Logical Operator8/1 -> Switch4/2
  Switch2/1 -> Logical Operator6/1, Timer1/2, SR_Latch1/2(reset)
  DTC_Couter/1 -> SR_Latch4/1
  DTC_Couter/2 -> Data Type Conversion1/1
  Constant40/1 -> Test Detection Criteria/3
  [task_time_s] -> Timer1/3
  Timer1/1 -> Equal5/1
  Constant/1 -> Equal1/2
  Equal1/1 -> Logical Operator5/2
  Logical Operator4/1 -> Logical Operator5/1
  VPMM_PowerUpFault_enum/1 -> Equal1/1
  Logical Operator5/1 -> [VDDM_MidLvSaChkChk_flg]
  VDDM_MidLvSaChkChk_flg/1 -> Logical Operator4/1
  DTC_clear_request/1 -> [DTC_clear_request]
  DTC_Info/1 -> VDDM_MidLvSaChkDTC_raw32/1  "VDDM_MidLvSaChkDTC_raw32"
  [VDDM_MidLvSaChkPass_flg] -> DTC_Info/2
  [VDDM_MidLvSaChkCFS_flg] -> DTC_Info/3
  [VDDM_MidLvSaChkCFS_flg] -> SR_Latch3/2
  [VDDM_MidLvSaChkDet_flg] -> DTC_Info/1
  Constant38/1 -> Test Detection Criteria/4
  [DTC_clear_request] -> DTC_Info/4
  VPMM_PowerUpState_enum/1 -> [VPMM_PowerUpState_enum]
  Constant2/1 -> Switch2/1
  Constant1/1 -> Equal2/2
  [VPMM_PowerUpState_enum] -> Equal2/1

== system ddm/DDM/DDM/PMM/power up and power down/OBC ready for precharge fail ==
  note: Diagnostics and Fault Handling
  note: Fail Safe Operation During Failure Detection
  note: Release Condition After Failure Decision
  note: Fail Safe Operation After Failure Decision
  note: Test Detection Criteria
  note: Test Pass Criteria
  note: Release Condition During Failure Detection
  task_time_s : Inport
  VPMM_PowerSta_enum : Inport  Port=2
  VPMM_PwrStaSW_enum : Inport  Port=3
  VPMM_HVChrgPreActionErrSta_enum : Inport  Port=4
  DTC_clear_request : Inport  Port=5
  Constant1 : Constant  Value=ENUM_PWRSTASW_OFFCLVCHRG
  Constant10 : Constant  Value=KDDM_OBC4PreDTC_cnt
  Constant11 : Constant  Value=KDDM_OBC4PrePassSW_flg
  Constant15 : Constant  Value=KDDM_OBC4PreCFSSW_flg
  Constant16 : Constant  Value=TRUE
  Constant17 : Constant  Value=KDDM_OBC4PrePassTO_s
  Constant18 : Constant  Value=ENUM_PWRSTASW_ONHVCHRG
  Constant19 : Constant  Value=ENUM_POWERSTA_OFF
  Constant2 : Constant  Value=ENUM_PWRSTASW_OFFCLVCHRG
  Constant20 : Constant  Value=KDDM_OBC4PreDFSSW_flg
  Constant{8,21,25,27} (4 alike) : Constant  Value=FALSE
  Constant23 : Constant  Value=TRUE
  Constant24 : Constant  Value=TRUE
  Constant26 : Constant  Value=ENUM_PWRSTASW_ON
  Constant3 : Constant  Value=ENUM_CHGPREACTERRSTA_OBCPRE
  Constant38 : Constant  Value=KDDM_OBC4PreDetTO_s
  Constant4 : Constant  Value=ENUM_PWRSTASW_ONHVCHRG
  Constant40 : Constant  Value=KDDM_OBC4PreDTC_cnt
  Constant43 : Constant  Value=KDDM_OBC4PrePassTO_s
  Constant44 : Constant  Value=KDDM_OBC4PreDetSW_flg
  Constant5 : Constant  Value=ENUM_PWRSTASW_ON
  Constant6 : Constant  Value=ENUM_PWRSTASW_OFFCHVCHRG
  Constant7 : Constant  Value=ENUM_PWRSTASW_OFFCHVCHRG
  DTC_Couter : hcu_lib/Basic_Blocks/DTC_Couter
  DTC_Info : hcu_lib/Basic_Blocks/DTC_Info
  Data Type Conversion1 : DataTypeConversion  OutDataTypeStr=uint8
  Equal{,1..4,6..9,24} (10 alike) : RelationalOperator  Operator===  OutDataTypeStr=boolean  RndMeth=Simplest
  Equal5 : RelationalOperator  OutDataTypeStr=boolean  RndMeth=Simplest
  Goto24 : Goto  Commented=on  GotoTag=VDDM_EDriveSysErrVCUErr_flg
  Logical Operator1 : Logic  Operator=OR  Inputs=4  AllPortsSameDT=off  OutDataTypeStr=boolean
  Logical Operator{12,15,18..19} (4 alike) : Logic  AllPortsSameDT=off  OutDataTypeStr=boolean
  Logical Operator2 : Logic  Operator=OR  Inputs=4  AllPortsSameDT=off  OutDataTypeStr=boolean
  Logical Operator3 : Logic  Operator=OR  AllPortsSameDT=off  OutDataTypeStr=boolean
  Logical Operator6 : Logic  Operator=NOT  AllPortsSameDT=off  OutDataTypeStr=boolean
  Logical Operator8 : Logic  Operator=OR  AllPortsSameDT=off  OutDataTypeStr=boolean
  Relay : Relay  OnSwitchValue=ONE_INT  OffSwitchValue=ZERO_INT
  SR_Latch1 : Subsystem  mask(SR_Latch){}
      mask help: SR latch function.
  SR_Latch3 : hcu_lib/Basic_Blocks/SR_Latch
  SR_Latch4 : hcu_lib/Basic_Blocks/SR_Latch
  Switch{,1..2,4..5} (5 alike) : Switch  Criteria=u2 ~= 0
  Test Detection Criteria : hcu_lib/Basic_Blocks/Test Detection Criteria
  Timer1 : hcu_lib/Basic_Blocks/Timer
  VDDM_OBC4PreDTC_raw32 : Outport
  wires:
  task_time_s/1 -> [task_time_s]
  VPMM_PwrStaSW_enum/1 -> [VPMM_PwrStaSW_enum]
  VPMM_PowerSta_enum/1 -> [VPMM_PowerSta_enum]
  Constant3/1 -> Equal24/2
  VPMM_HVChrgPreActionErrSta_enum/1 -> Equal24/1
  Equal24/1 -> [VDDM_OBC4PreChk_flg]  "VDDM_OBC4PreChk_flg"
  DTC_Couter/2 -> Data Type Conversion1/1
  [VPMM_PwrStaSW_enum] -> Equal8/1
  [task_time_s] -> Timer1/3
  DTC_Couter/1 -> SR_Latch4/1
  Constant40/1 -> Test Detection Criteria/3
  Constant7/1 -> Equal3/2
  Timer1/1 -> Equal5/1
  Relay/1 -> SR_Latch3/1
  Constant10/1 -> DTC_Couter/3
  [VDDM_OBC4PreDTC_cnt] -> Relay/1
  Constant24/1 -> Switch4/1
  [VDDM_OBC4PreCFSRls_flg] -> Logical Operator3/2
  Logical Operator6/1 -> Timer1/1
  SR_Latch1/1(latched) -> [VDDM_OBC4PrePass_flg]
  SR_Latch3/1 -> Logical Operator12/2
  Switch/1 -> Goto24/1
  [task_time_s] -> Test Detection Criteria/2
  Constant20/1 -> Logical Operator12/1
  Equal6/1 -> Logical Operator8/1
  Logical Operator12/1 -> [VDDM_OBC4PreDFS_flg]
  Logical Operator2/1 -> Switch5/2
  Constant15/1 -> Logical Operator18/2
  Test Detection Criteria/1 -> [VDDM_OBC4PreDet_flg]  "VDDM_OBC4PreDet_flg"
  Equal5/1 -> SR_Latch1/1(set)
  Constant21/1 -> Switch/3
  Logical Operator18/1 -> [VDDM_OBC4PreCFS_flg]
  [VPMM_PwrStaSW_enum] -> Equal/1
  Constant18/1 -> Equal8/2
  [VDDM_OBC4PreChk_flg] -> Switch5/1
  Switch4/1 -> [VDDM_OBC4PreCFSRls_flg]
  Constant19/1 -> Equal6/2
  [VDDM_OBC4PreCFS_flg] -> Switch/2
  Constant26/1 -> Equal/2
  Data Type Conversion1/1 -> [VDDM_OBC4PreDTC_cnt]  "VDDM_OBC4PreDTC_cnt"
  Constant44/1 -> Logical Operator19/2
  Constant16/1 -> Switch/1
  Switch1/1 -> Logical Operator6/1, Timer1/2
  Constant25/1 -> Switch4/3
  Logical Operator8/1 -> Switch4/2
  [VDDM_OBC4PreCFSRls_flg] -> SR_Latch4/2
  Constant43/1 -> Timer1/4
  [VDDM_OBC4PrePass_flg] -> Logical Operator3/1
  Constant27/1 -> Switch5/3
  Logical Operator19/1 -> DTC_Couter/1
  Constant11/1 -> Logical Operator15/2
  [VPMM_PowerSta_enum] -> Equal6/1
  [VPMM_PwrStaSW_enum] -> Equal3/1
  [VDDM_OBC4PreDet_flg] -> Logical Operator19/1
  Logical Operator3/1 -> Logical Operator15/1
  Constant17/1 -> Equal5/2
  Logical Operator15/1 -> DTC_Couter/2
  SR_Latch4/1 -> Logical Operator18/1
  Constant23/1 -> Switch1/3
  [DTC_clear_request] -> Logical Operator8/2
  DTC_clear_request/1 -> [DTC_clear_request]
  [VPMM_PwrStaSW_enum] -> Equal1/1
  Constant1/1 -> Equal1/2
  Equal8/1 -> Logical Operator2/4
  Equal1/1 -> Logical Operator2/3
  Equal/1 -> Logical Operator2/2
  Equal3/1 -> Logical Operator2/1
  Constant2/1 -> Equal4/2
  [VPMM_PwrStaSW_enum] -> Equal4/1
  Equal7/1 -> Logical Operator1/1
  Equal2/1 -> Logical Operator1/2
  Equal4/1 -> Logical Operator1/3
  Equal9/1 -> Logical Operator1/4
  [VPMM_PwrStaSW_enum] -> Equal7/1
  [VDDM_OBC4PreChk_flg] -> Switch1/1
  Constant5/1 -> Equal2/2
  Logical Operator1/1 -> Switch1/2
  [VPMM_PwrStaSW_enum] -> Equal2/1
  Constant6/1 -> Equal7/2
  Constant4/1 -> Equal9/2
  [VPMM_PwrStaSW_enum] -> Equal9/1
  DTC_Info/1 -> VDDM_OBC4PreDTC_raw32/1  "VDDM_OBC4PreDTC_raw32"
  [VDDM_OBC4PrePass_flg] -> DTC_Info/2
  [VDDM_OBC4PreCFS_flg] -> DTC_Info/3
  [VDDM_OBC4PreCFS_flg] -> SR_Latch3/2
  [VDDM_OBC4PreDet_flg] -> DTC_Info/1
  Constant38/1 -> Test Detection Criteria/4
  [DTC_clear_request] -> DTC_Info/4
  Switch5/1 -> [VDDM_xxx_flg], Switch2/3
  [DTC_clear_request] -> Switch2/2
  Constant8/1 -> Switch2/1
  Switch2/1 -> Test Detection Criteria/1
  [VDDM_xxx_flg] -> SR_Latch1/2(reset)
